simulink model "REHROBNL"  (R2024a)
settings: Solver=FixedStepAuto  StartTime=0.0  StopTime=10  FixedStep=dt  MaxStep=1e-4  RelTol=1e-5
values from neighbouring files (symbols this model uses):
  kd = [10 0;0 10]    [RehabilitationRobotDecouplingBased_Final_version_Vlad.m]
  kp = [400 0 ;0 600]    [RehabilitationRobotDecouplingBased_Final_version_Vlad.m]
  r1f = 4.0*pi/18    (= 0.698131700798)    [RehabilitationRobotDecouplingBased_Final_version_Vlad.m]
  r1i = 0    [RehabilitationRobotDecouplingBased_Final_version_Vlad.m]
  r1m = 4.5*pi/18    (= 0.785398163397)    [RehabilitationRobotDecouplingBased_Final_version_Vlad.m]
  r2f = 4.0*pi/18    (= 0.698131700798)    [RehabilitationRobotDecouplingBased_Final_version_Vlad.m]
  r2i = 0    [RehabilitationRobotDecouplingBased_Final_version_Vlad.m]
  r2m = 7.0*pi/18    (= 1.2217304764)    [RehabilitationRobotDecouplingBased_Final_version_Vlad.m]
  t1f = t1m + 2.0    (= 4.5)    [RehabilitationRobotDecouplingBased_Final_version_Vlad.m]
  t1i = 0    [RehabilitationRobotDecouplingBased_Final_version_Vlad.m]
  t1m = t1i + 2.5    (= 2.5)    [RehabilitationRobotDecouplingBased_Final_version_Vlad.m]
  t2f = t2m + 2.0    (= 4.5)    [RehabilitationRobotDecouplingBased_Final_version_Vlad.m]
  t2i = 0    [RehabilitationRobotDecouplingBased_Final_version_Vlad.m]
  t2m = t2i + 2.5    (= 2.5)    [RehabilitationRobotDecouplingBased_Final_version_Vlad.m]
  y1_0 = 0    [RehabilitationRobotDecouplingBased_Final_version_Vlad.m]
  y1_dot_0 = 0    [RehabilitationRobotDecouplingBased_Final_version_Vlad.m]
  y2_0 = 0    [RehabilitationRobotDecouplingBased_Final_version_Vlad.m]
  y2_dot_0 = 0    [RehabilitationRobotDecouplingBased_Final_version_Vlad.m]
settings Model: Creator=KorogluH  LastModifiedBy=31629
settings SolverCC: AlgebraicLoopSolver=TrustRegion
settings DebuggingCC: UnconnectedInputMsg=warning  UnconnectedOutputMsg=warning  UnconnectedLineMsg=warning
settings ModelReferenceCC: EnableRefExpFcnMdlSchedulingChecks=on
settings SFSimCC: CustomCodeUndefinedFunction=UseInterfaceOnly
settings RTWCC: GPUComputeCapability=3.5  DLArmComputeVersion=19.05

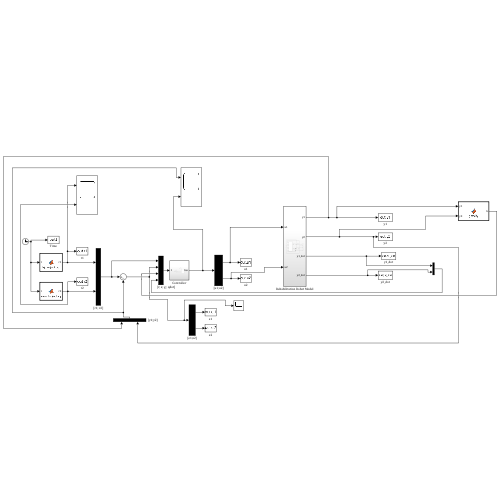
[thumbnail: Simulink's stored preview of the top-level diagram]
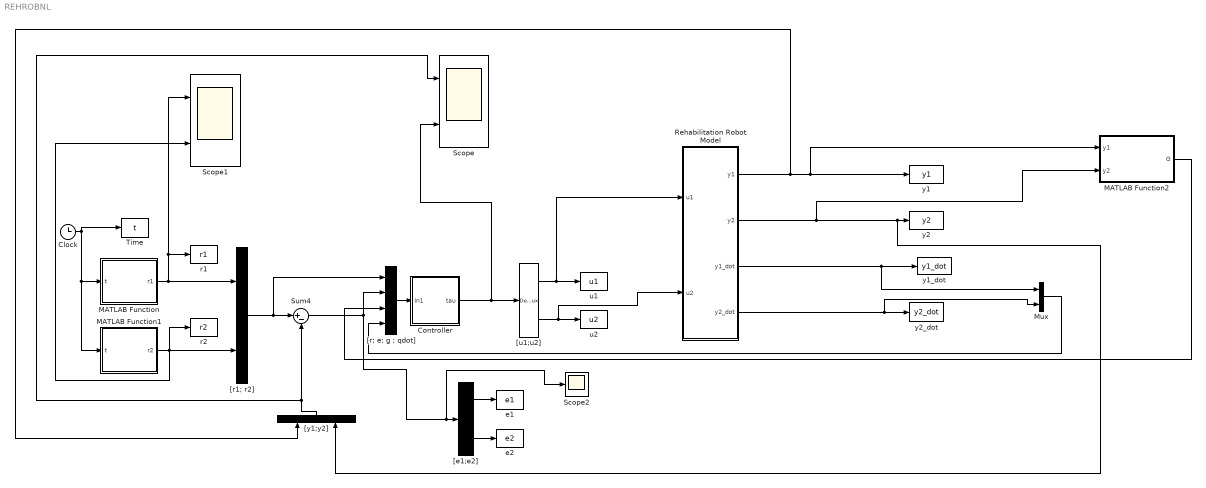
== system REHROBNL ==
  "               [r; e; g ; qdot]" : Mux  Inputs=[2 2 2 2]
  Clock : Clock
  Controller : Subsystem
  MATLAB Function : MATLAB Function  TreatAsAtomicUnit=on
  MATLAB Function1 : MATLAB Function  TreatAsAtomicUnit=on
  MATLAB Function2 : MATLAB Function  TreatAsAtomicUnit=on
  Mux : Mux  Inputs=2
  Rehabilitation Robot Model : Subsystem
  Scope : Scope  NumInputPorts=2
  Scope1 : Scope  NumInputPorts=2
  Scope2 : Scope
  Sum4 : Sum  Inputs=|+-
  Time : ToWorkspace  VariableName=t  SampleTime=-1
      settings: Save2DSignal=2-D array (concatenate along first dimension)
  "[e1;e2]" : Demux  Outputs=[1 1]
  "[r1; r2]" : Mux  Inputs=[1 1]
  "[u1;u2]" : Demux  Outputs=[1 1]
  "[y1;y2]" : Mux  Inputs=[1 1]
  e1 : ToWorkspace  VariableName=e1  SampleTime=-1
  e2 : ToWorkspace  VariableName=e2  SampleTime=-1
  r1 : ToWorkspace  VariableName=r1  SampleTime=-1
  r2 : ToWorkspace  VariableName=r2  SampleTime=-1
  u1 : ToWorkspace  VariableName=u1  SampleTime=-1
      settings: Save2DSignal=2-D array (concatenate along first dimension)
  u2 : ToWorkspace  VariableName=u2  SampleTime=-1
      settings: Save2DSignal=2-D array (concatenate along first dimension)
  y1 : ToWorkspace  VariableName=y1  SampleTime=-1
      settings: Save2DSignal=2-D array (concatenate along first dimension)
  y1_dot : ToWorkspace  VariableName=y1_dot  SampleTime=-1
      settings: Save2DSignal=2-D array (concatenate along first dimension)
  y2 : ToWorkspace  VariableName=y2  SampleTime=-1
      settings: Save2DSignal=2-D array (concatenate along first dimension)
  y2_dot : ToWorkspace  VariableName=y2_dot  SampleTime=-1
      settings: Save2DSignal=2-D array (concatenate along first dimension)
  wires:
  Clock/1 -> Time/1, MATLAB Function1/1(t), MATLAB Function/1(t)
  MATLAB Function/1(r1) -> "[r1; r2]"/1, Scope1/1, r1/1
  "[r1; r2]"/1 -> "               [r; e; g ; qdot]"/1, Sum4/1
  MATLAB Function1/1(r2) -> r2/1, Scope1/2, "[r1; r2]"/2
  "[u1;u2]"/2 -> Rehabilitation Robot Model/2(u2), u2/1
  Rehabilitation Robot Model/1(y1) -> y1/1, MATLAB Function2/1(y1), "[y1;y2]"/1
  Rehabilitation Robot Model/3(y1_dot) -> Mux/1, y1_dot/1
  "[u1;u2]"/1 -> Rehabilitation Robot Model/1(u1), u1/1
  "[y1;y2]"/1 -> Sum4/2, Scope/1
  Sum4/1 -> Scope2/1, "[e1;e2]"/1, "               [r; e; g ; qdot]"/2
  Rehabilitation Robot Model/4(y2_dot) -> Mux/2, y2_dot/1
  "[e1;e2]"/1 -> e1/1
  "[e1;e2]"/2 -> e2/1
  Rehabilitation Robot Model/2(y2) -> y2/1, "[y1;y2]"/2, MATLAB Function2/2(y2)
  Controller/1(tau) -> Scope/2, "[u1;u2]"/1
  "               [r; e; g ; qdot]"/1 -> Controller/1(In1)
  MATLAB Function2/1(G) -> "               [r; e; g ; qdot]"/3
  Mux/1 -> "               [r; e; g ; qdot]"/4

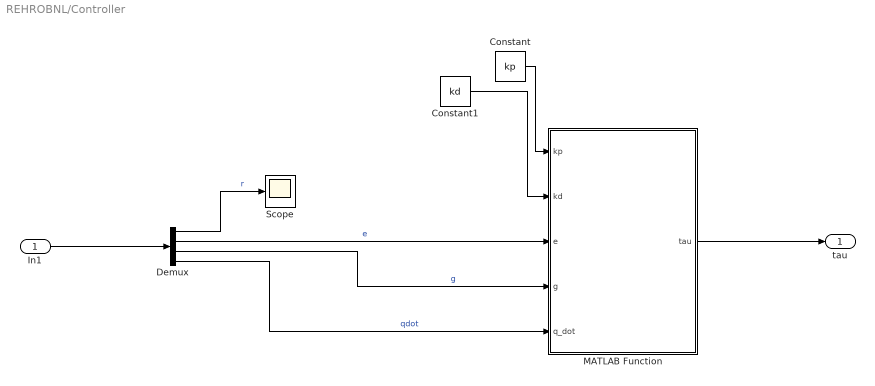
== system REHROBNL/Controller ==
  In1 : Inport
  Constant : Constant  Value=kp
  Constant1 : Constant  Value=kd
  Demux : Demux
  MATLAB Function : MATLAB Function  TreatAsAtomicUnit=on
  Scope : Scope
  tau : Outport
  wires:
  MATLAB Function/1(tau) -> tau/1
  In1/1 -> Demux/1
  Demux/2 -> MATLAB Function/3(e)  "e"
  Demux/3 -> MATLAB Function/4(g)  "g"
  Constant/1 -> MATLAB Function/1(kp)
  Constant1/1 -> MATLAB Function/2(kd)
  Demux/4 -> MATLAB Function/5(q_dot)  "qdot"
  Demux/1 -> Scope/1  "r"

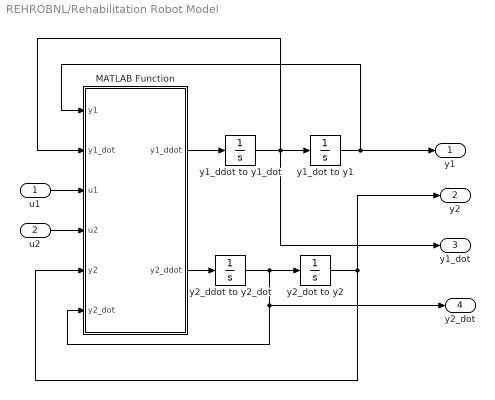
== system REHROBNL/Rehabilitation Robot Model ==
  u1 : Inport
  u2 : Inport  Port=2
  MATLAB Function : MATLAB Function  TreatAsAtomicUnit=on
  y1_ddot to y1_dot : Integrator  InitialCondition=y1_dot_0
  y1_dot to y1 : Integrator  InitialCondition=y1_0
  y2_ddot to y2_dot : Integrator  InitialCondition=y2_dot_0
  y2_dot to y2 : Integrator  InitialCondition=y2_0
  y1 : Outport
  y2 : Outport  Port=2
  y1_dot : Outport  Port=3
  y2_dot : Outport  Port=4
  wires:
  y1_ddot to y1_dot/1 -> y1_dot/1, MATLAB Function/2(y1_dot), y1_dot to y1/1
  y2_ddot to y2_dot/1 -> MATLAB Function/6(y2_dot), y2_dot/1, y2_dot to y2/1
  y1_dot to y1/1 -> MATLAB Function/1(y1), y1/1
  y2_dot to y2/1 -> y2/1, MATLAB Function/5(y2)
  MATLAB Function/1(y1_ddot) -> y1_ddot to y1_dot/1
  MATLAB Function/2(y2_ddot) -> y2_ddot to y2_dot/1
  u1/1 -> MATLAB Function/3(u1)
  u2/1 -> MATLAB Function/4(u2)

== matlab function REHROBNL/MATLAB Function1 ==
  data: t input; r2 output; t2i parameter; t2m parameter; t2f parameter; r2i parameter; r2m parameter; r2f parameter
function r2 = kneetrajectory(t, t2i, t2m, t2f, r2i, r2m, r2f)

if t<t2i
    r2 = r2i;
elseif t < t2m
    r2 = r2i + (r2m-r2i)*((t-t2i)/(t2m-t2i) - sin(2*pi*(t-t2i)/(t2m-t2i))/(2*pi));
elseif t < t2f
    r2 = r2m + (r2f-r2m)*((t-t2m)/(t2f-t2m) - sin(2*pi*(t-t2m)/(t2f-t2m))/(2*pi));
else
    r2 = r2f;
end

== matlab function REHROBNL/MATLAB Function ==
  data: t input; r1 output; t1i parameter; t1m parameter; t1f parameter; r1i parameter; r1m parameter; r1f parameter
function r1 = hiptrajectory(t, t1i, t1m, t1f, r1i, r1m, r1f)

if t<t1i
    r1 = r1i;
elseif t < t1m
    r1 = r1i + (r1m-r1i)*((t-t1i)/(t1m-t1i) - sin(2*pi*(t-t1i)/(t1m-t1i))/(2*pi));
elseif t < t1f
    r1 = r1m + (r1f-r1m)*((t-t1m)/(t1f-t1m) - sin(2*pi*(t-t1m)/(t1f-t1m))/(2*pi));
else
    r1 = r1f;
end

== matlab function REHROBNL/Controller/MATLAB Function ==
  data: kp input; kd input; e input; g input; q_dot input; tau output
function tau = controller(kp,kd,e,g,q_dot)


tau = kp*(e) - kd*q_dot + g;

== matlab function REHROBNL/Rehabilitation Robot Model/MATLAB Function ==
  data: y1 input; y1_dot input; u1 input; u2 input; y1_ddot output; y2 input; y2_dot input; y2_ddot output
function [y1_ddot,y2_ddot] = rehrobot(y1,y1_dot,u1,u2,y2,y2_dot)

%% Input and States
tau      = [u1    ; u2    ];
y      = [y1    ; y2    ];
y_dot  = [y1_dot; y2_dot];

%% Parameters
m1 = 4.0  ; m2 = 3    ;
M1 = 9.847; M2 = 3.086;
M3 = 1.93 ; g  = 9.8  ;
l1 = 0.496; l2 = 0.396;
L1 = 0.265; L2 = 0.229;
I1 = 0.164; I2 = 0.028;
b1 = 1e-1 ; b2 = 1e-1 ;



J11 = (m1+M1)*(L1)^2+(m2+M2)*(l1)^2+(m2+M2)*(L2)^2+2*(m2+M2)*l1*L2*cos(y(2))+M3*(l1)^2+M3*(l2)^2+2*M3*l1*l2*cos(y(2))+I1;
J12 = -(m2+M2)*(L2)^2-(m2+M2)*l1*L2*cos(y(2))-M3*(l2)^2-M3*l1*l2*cos(y(2));
J21 = J12;
J22 = (m2+M2)*(L2)^2+M3*(l2)^2+I2;
%Inertia matrix
J = [J11 J12; J21 J22];

B11 =-2*(m2+M2)*l1*L2*y_dot(2)*sin(y(2))-2*M3*l1*l2*y_dot(2)*sin(y(2))+b1;
B12 = (m2+M2)*l1*L2*y_dot(2)*sin(y(2))+M3*l1*l2*y_dot(2)*sin(y(2));
B21 = (m2+M2)*l1*L2*y_dot(1)*sin(y(2))+M3*l1*l2*y_dot(1)*sin(y(2));
B22 = b2;
%Coriolis matrix
B = [B11 B12; B21 B22];

G1 = (m1+M1)*g*L1*sin(y(1))+(m2+M2)*g*l1*sin(y(1))+(m2+M2)*g*L2*sin(y(1)-y(2))+M3*g*l1*sin(y(1))+M3*g*l2*sin(y(1)-y(2));
G2 = -((m2+M2)*g*L2*sin(y(1)-y(2))+(M3*g*l2*sin(y(1)-y(2))));
%gravity vector
G  = [G1;G2];

y_ddot = tau.*inv(J) - G.*inv(J) - B.*inv(J).*y_dot;

y1_ddot = y_ddot(1);
y2_ddot = y_ddot(2);

== matlab function REHROBNL/MATLAB Function2 ==
  data: y1 input; G output; y2 input
function G = gravity(y1,y2)

%% Input and States

y      = [y1    ; y2    ];

%% Parameters
m1 = 4.0  ; m2 = 3    ;
M1 = 9.847; M2 = 3.086;
M3 = 1.93 ; g  = 9.8  ;
l1 = 0.496; l2 = 0.396;
L1 = 0.265; L2 = 0.229;
I1 = 0.164; I2 = 0.028;
b1 = 1e-1 ; b2 = 1e-1 ;

G1 = (m1+M1)*g*L1*sin(y(1))+(m2+M2)*g*l1*sin(y(1))+(m2+M2)*g*L2*sin(y(1)-y(2))+M3*g*l1*sin(y(1))+M3*g*l2*sin(y(1)-y(2));
G2 = -((m2+M2)*g*L2*sin(y(1)-y(2))+(M3*g*l2*sin(y(1)-y(2))));
%gravity vector
G  = [G1;G2];
